simulink model "model"  (Simulink 8.7)
settings: Solver=FixedStepAuto  StartTime=0.0  StopTime=25  FixedStep=0.001  RelTol=1e-3
libraries: simulink x2
settings Model: Creator=farid_000  LastModifiedBy=TheChosenOne
settings DataIOCC: ExternalInput=p , i , d  LimitDataPoints=off  SaveFormat=Dataset  SaveOutput=off  SignalLogging=off  DSMLogging=off  SaveTime=off
settings DebuggingCC: UnderspecifiedInitializationDetection=Simplified  MergeDetectMultiDrivingBlocksExec=error  AllowSymbolicDim=off
settings HardwareCC: ProdBitPerPointer=64  ProdLargestAtomicFloat=Float  ProdIntDivRoundTo=Zero  ProdEndianess=LittleEndian  ProdWordSize=64  ProdHWDeviceType=Intel->x86-64 (Windows64)
settings GRTTargetCC: GeneratePreprocessorConditionals=Use local settings
settings ConfigComp: CovModelRefEnable=off

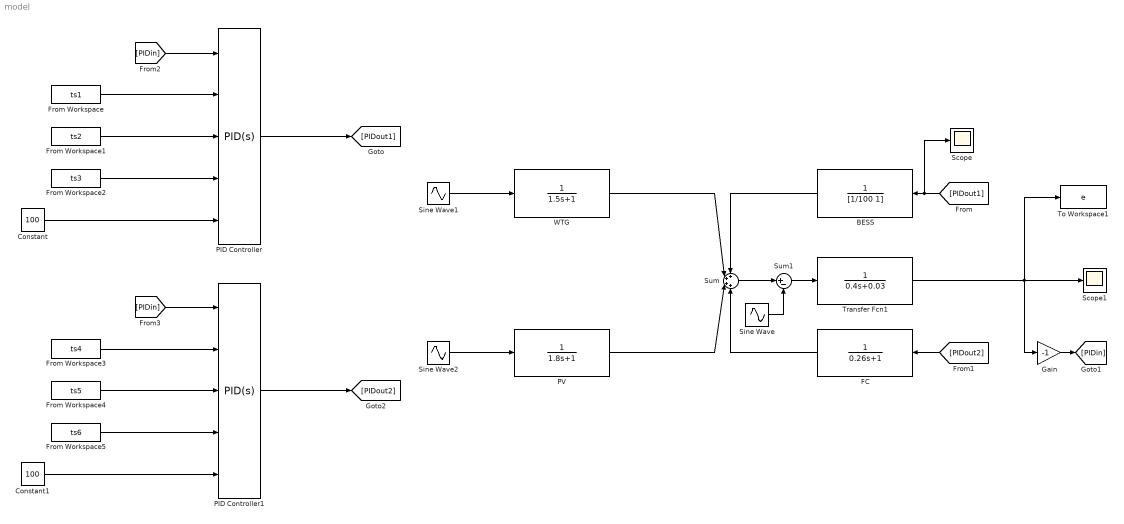
== system model ==
  BESS : TransferFcn  Denominator=[1/100 1]
  Constant : Constant  Value=100
  Constant1 : Constant  Value=100
  FC : TransferFcn  Denominator=[0.26 1]
  From Workspace : FromWorkspace  VariableName=ts1  SampleTime=0
  From Workspace1 : FromWorkspace  VariableName=ts2  SampleTime=0
  From Workspace2 : FromWorkspace  VariableName=ts3  SampleTime=0
  From Workspace3 : FromWorkspace  VariableName=ts4  SampleTime=0
  From Workspace4 : FromWorkspace  VariableName=ts5  SampleTime=0
  From Workspace5 : FromWorkspace  VariableName=ts6  SampleTime=0
  Gain : Gain  Gain=-1
  PID Controller : simulink/Continuous/PID Controller  Controller=PID  TimeDomain=Continuous-time  SampleTime=-1  IntegratorMethod=Forward Euler  FilterMethod=Forward Euler  Form=Parallel  UseFilter=on  ControllerParametersSource=external  P=1  I=1  D=0  N=100  InitialConditionSource=internal  InitialConditionForIntegrator=0  InitialConditionForFilter=0  ExternalReset=none  ZeroCross=off  LimitOutput=on  UpperSaturationLimit=10  LowerSaturationLimit=-10  LinearizeAsGain=on  AntiWindupMode=none  Kb=1  TrackingMode=off  Kt=1  PParamMin=[]  PParamMax=[]  IParamMin=[]  IParamMax=[]  DParamMin=[]  DParamMax=[]  NParamMin=[]  NParamMax=[]  KbParamMin=[]  KbParamMax=[]  KtParamMin=[]  KtParamMax=[]  POutMin=[]  POutMax=[]  IOutMin=[]  IOutMax=[]  DOutMin=[]  DOutMax=[]  NOutMin=[]  NOutMax=[]  KbOutMin=[]  KbOutMax=[]  KtOutMin=[]  KtOutMax=[]  IntegratorOutMin=[]  IntegratorOutMax=[]  FilterOutMin=[]  FilterOutMax=[]  SumOutMin=[]  SumOutMax=[]  SumI1OutMin=[]  SumI1OutMax=[]  SumI2OutMin=[]  SumI2OutMax=[]  SumI3OutMin=[]  SumI3OutMax=[]  SumDOutMin=[]  SumDOutMax=[]  SaturationOutMin=[]  SaturationOutMax=[]  IntegratorContinuousStateAttributes=''  IntegratorStateMustResolveToSignalObject=off  IntegratorRTWStateStorageClass=Auto  FilterContinuousStateAttributes=''  FilterStateMustResolveToSignalObject=off  FilterRTWStateStorageClass=Auto  DifferentiatorICPrevScaledInput=0  DifferentiatorOutMin=[]  DifferentiatorOutMax=[]
  PID Controller1 : simulink/Continuous/PID Controller  Controller=PID  TimeDomain=Continuous-time  SampleTime=-1  IntegratorMethod=Forward Euler  FilterMethod=Forward Euler  Form=Parallel  UseFilter=on  ControllerParametersSource=external  P=1  I=1  D=0  N=100  InitialConditionSource=internal  InitialConditionForIntegrator=0  InitialConditionForFilter=0  ExternalReset=none  ZeroCross=off  LimitOutput=on  UpperSaturationLimit=10  LowerSaturationLimit=-10  LinearizeAsGain=on  AntiWindupMode=none  Kb=1  TrackingMode=off  Kt=1  PParamMin=[]  PParamMax=[]  IParamMin=[]  IParamMax=[]  DParamMin=[]  DParamMax=[]  NParamMin=[]  NParamMax=[]  KbParamMin=[]  KbParamMax=[]  KtParamMin=[]  KtParamMax=[]  POutMin=[]  POutMax=[]  IOutMin=[]  IOutMax=[]  DOutMin=[]  DOutMax=[]  NOutMin=[]  NOutMax=[]  KbOutMin=[]  KbOutMax=[]  KtOutMin=[]  KtOutMax=[]  IntegratorOutMin=[]  IntegratorOutMax=[]  FilterOutMin=[]  FilterOutMax=[]  SumOutMin=[]  SumOutMax=[]  SumI1OutMin=[]  SumI1OutMax=[]  SumI2OutMin=[]  SumI2OutMax=[]  SumI3OutMin=[]  SumI3OutMax=[]  SumDOutMin=[]  SumDOutMax=[]  SaturationOutMin=[]  SaturationOutMax=[]  IntegratorContinuousStateAttributes=''  IntegratorStateMustResolveToSignalObject=off  IntegratorRTWStateStorageClass=Auto  FilterContinuousStateAttributes=''  FilterStateMustResolveToSignalObject=off  FilterRTWStateStorageClass=Auto  DifferentiatorICPrevScaledInput=0  DifferentiatorOutMin=[]  DifferentiatorOutMax=[]
  PV : TransferFcn  Denominator=[1.8 1]
  Scope : Scope
  Scope1 : Scope
  Sine Wave : Sin  SampleTime=0
  Sine Wave1 : Sin  SampleTime=0
  Sine Wave2 : Sin  SampleTime=0
  Sum : Sum  Inputs=++++
  Sum1 : Sum  Inputs=|+-
  To Workspace1 : ToWorkspace  VariableName=e  SampleTime=-1
  Transfer Fcn1 : TransferFcn  Denominator=[0.4 0.03]
  WTG : TransferFcn  Denominator=[1.5 1]
  wires:
  From Workspace/1 -> PID Controller/2
  From Workspace2/1 -> PID Controller/4
  Constant/1 -> PID Controller/5
  From Workspace1/1 -> PID Controller/3
  Sum/1 -> Sum1/1
  WTG/1 -> Sum/2
  PV/1 -> Sum/3
  BESS/1 -> Sum/1
  FC/1 -> Sum/4
  Sum1/1 -> Transfer Fcn1/1
  Transfer Fcn1/1 -> Scope1/1, To Workspace1/1, Gain/1
  From Workspace3/1 -> PID Controller1/2
  From Workspace5/1 -> PID Controller1/4
  Constant1/1 -> PID Controller1/5
  From Workspace4/1 -> PID Controller1/3
  PID Controller/1 -> [PIDout1]
  [PIDout1] -> Scope/1, BESS/1
  [PIDout2] -> FC/1
  [PIDin] -> PID Controller/1
  [PIDin] -> PID Controller1/1
  PID Controller1/1 -> [PIDout2]
  Sine Wave1/1 -> WTG/1
  Sine Wave2/1 -> PV/1
  Sine Wave/1 -> Sum1/2
  Gain/1 -> [PIDin]
